simulink model "sim_sistema_obs_tf_1"  (Simulink 7.5)
settings: Solver=ode3  StartTime=0.0  StopTime=25  FixedStep=1e-4  RelTol=1e-3
values from neighbouring files (symbols this model uses):
  A = sys.a    [exemplo_obs.m]
  B = sys.b    [exemplo_obs.m]
  K = acker(A,B,J)    [exemplo_obs.m]
undefined symbols (not defined in the file or in its folder): den, num
settings Model: Creator=taniel.franklin  LastModifiedBy=taniel.franklin

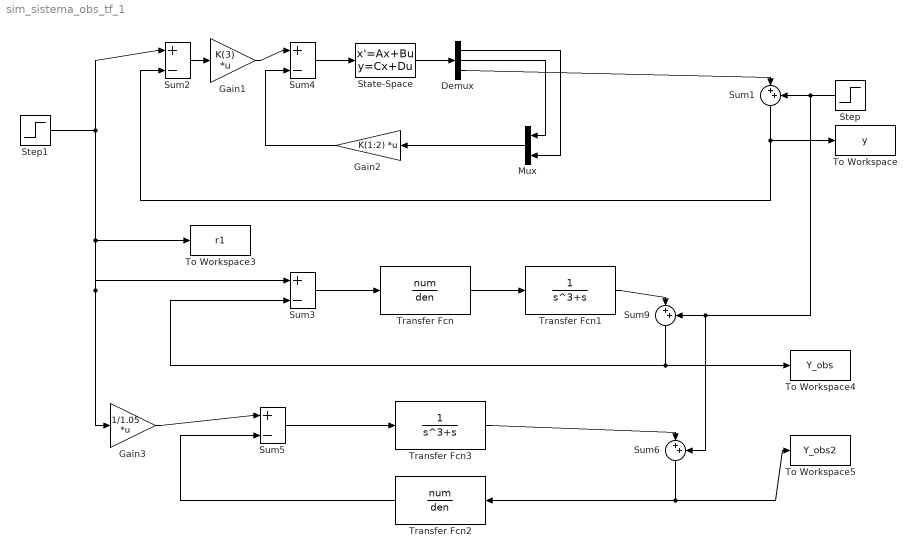
== system sim_sistema_obs_tf_1 ==
  Demux : Demux  Outputs=3
  Gain1 : Gain  Gain=K(3)  Multiplication=Matrix(K*u)  ParameterDataType=fixdt(1, 16)  ParameterScaling=2^0  OutDataType=fixdt(1, 16)  OutScaling=2^0
  Gain2 : Gain  Gain=K(1:2)  Multiplication=Matrix(K*u)  ParameterDataType=fixdt(1, 16)  ParameterScaling=2^0  OutDataType=fixdt(1, 16)  OutScaling=2^0
  Gain3 : Gain  Gain=1/1.05  Multiplication=Matrix(K*u)  ParameterDataType=fixdt(1, 16)  ParameterScaling=2^0  OutDataType=fixdt(1, 16)  OutScaling=2^0
  Mux : Mux  Inputs=2
  State-Space : StateSpace  A=A  B=B  C=eye(3)  D=[0;0;0]
  Step : Step  Time=12  After=0.2  SampleTime=0
  Step1 : Step  Time=0.3  SampleTime=0
  Sum1 : Sum  Inputs=|++  OutDataType=fixdt(1, 16)  OutScaling=2^0
  Sum{2..5} (4 alike) : Sum  Inputs=|+-  OutDataType=fixdt(1, 16)  OutScaling=2^0
  Sum6 : Sum  Inputs=|++  OutDataType=fixdt(1, 16)  OutScaling=2^0
  Sum9 : Sum  Inputs=|++  OutDataType=fixdt(1, 16)  OutScaling=2^0
  To Workspace : ToWorkspace  VariableName=y  SampleTime=-1  SaveFormat=Structure With Time
  To Workspace3 : ToWorkspace  VariableName=r1  SampleTime=-1  SaveFormat=Structure With Time
  To Workspace4 : ToWorkspace  VariableName=Y_obs  SampleTime=-1  SaveFormat=Structure With Time
  To Workspace5 : ToWorkspace  VariableName=Y_obs2  SampleTime=-1  SaveFormat=Structure With Time
  Transfer Fcn : TransferFcn  Numerator=num  Denominator=den
  Transfer Fcn1 : TransferFcn  Numerator=1  Denominator=[1 0 1 0]
  Transfer Fcn2 : TransferFcn  Numerator=num  Denominator=den
  Transfer Fcn3 : TransferFcn  Numerator=1  Denominator=[1 0 1 0]
  wires:
  State-Space/1 -> Demux/1
  Transfer Fcn1/1 -> Sum9/1
  Sum9/1 -> Sum3/2, To Workspace4/1
  Mux/1 -> Gain2/1
  Sum3/1 -> Transfer Fcn/1
  Step1/1 -> Sum2/1, To Workspace3/1, Sum3/1, Gain3/1
  Transfer Fcn/1 -> Transfer Fcn1/1
  Demux/3 -> Sum1/1
  Sum1/1 -> To Workspace/1, Sum2/2
  Sum2/1 -> Gain1/1
  Sum4/1 -> State-Space/1
  Gain2/1 -> Sum4/2
  Gain1/1 -> Sum4/1
  Transfer Fcn3/1 -> Sum6/1
  Sum6/1 -> To Workspace5/1, Transfer Fcn2/1
  Sum5/1 -> Transfer Fcn3/1
  Transfer Fcn2/1 -> Sum5/2
  Gain3/1 -> Sum5/1
  Step/1 -> Sum1/2, Sum9/2, Sum6/2
  Demux/2 -> Mux/1
  Demux/1 -> Mux/2
